simulink model "ddcnco"  (Simulink 6.1)
settings: Solver=FixedStepDiscrete  SolverMode=SingleTasking  StartTime=0.0  StopTime=20544/69.333e6  RelTol=1e-3
values from neighbouring files (symbols this model uses):
  D = [0 : 1/1E3 : 10E-3 ; 0.8.^(0:10)]'    [waveformdemo.m]
libraries: simulink x6, dspsnks4 x1, dspsigops x1, dspindex x1
settings Model: MinMaxOverflowLogging=OverflowOnly  Creator=The MathWorks Inc.  LastModifiedBy=pjp  ExtModeAutoUpdateStatusClock=off  ProdHWDeviceType=ASIC/FPGA
settings DataIOCC: LimitDataPoints=off  SaveOutput=off  SignalLogging=off  SaveTime=off  SignalLoggingName=sigsOut
settings OptimizationCC: InlineParams=on  BufferReusableBoundary=off
settings DebuggingCC: CheckExecutionContextPreStartOutputMsg=on  CheckExecutionContextRuntimeOutputMsg=on  IntegerOverflowMsg=none  ParameterPrecisionLossMsg=none  BusObjectLabelMismatch=off
settings HardwareCC: ProdHWDeviceType=ASIC/FPGA

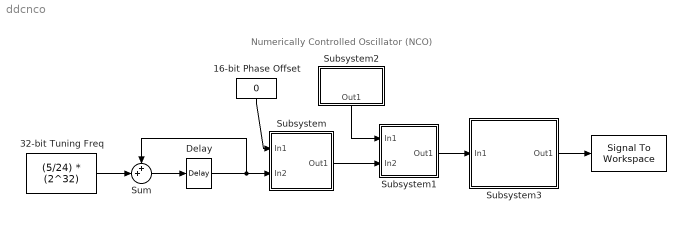
== system ddcnco ==
  note: Numerically Controlled Oscillator (NCO)
  "  " : dspsnks4/Signal To Workspace  VariableName=nco_nodither  FrameMode=Concatenate frames (2-D array)
      settings: AttributesFormatString=\n  Decimation=1  FixptAsFi=off
  16-bit Phase Offset : Constant  Orientation=down  Value=0  OutDataTypeMode=Specify via dialog  OutDataType=ufix(16)  OutScaling=2^-0  SampleTime=1/69.333e6
  32-bit Tuning Freq : Constant  Value=(5/24) * (2^32)  OutDataTypeMode=Specify via dialog  OutDataType=ufix(32)  OutScaling=2^-0  SampleTime=1/69.333e6
  Delay : dspsigops/Delay  dly_unit=Samples  delay=1  ic_detail=off  dif_ic_for_ch=off  dif_ic_for_dly=off  ic=0  reset_popup=None
  Subsystem : Subsystem
      mask Display: disp(['Sum and\nretain\n23 MSBs'])
  Subsystem1 : Subsystem
      mask Display: disp('Sum and\nretain\n18 MSBs')
  Subsystem2 : Subsystem  Orientation=down
      mask Display: disp(['Dither' 10 'Generator'])
  Subsystem3 : Subsystem
      mask Display: disp(['Sine/Cosine\nLookup'])
  Sum : Sum  Inputs=++|  OutDataTypeMode=uint32  RndMeth=Nearest
  wires:
  Delay/1 -> Sum/1, Subsystem/2(In2)
  Sum/1 -> Delay/1
  Subsystem1/1(Out1) -> Subsystem3/1(In1)
  Subsystem3/1(Out1) -> "  "/1
  16-bit Phase Offset/1 -> Subsystem/1(In1)
  Subsystem2/1(Out1) -> Subsystem1/1(In1)
  Subsystem/1(Out1) -> Subsystem1/2(In2)
  32-bit Tuning Freq/1 -> Sum/2

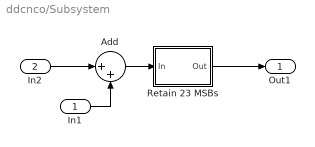
== system ddcnco/Subsystem ==
  In1 : Inport  Port=1  LatchInput=off
  In2 : Inport  Port=2  LatchInput=off
  Add : Sum  Inputs=|++  OutDataTypeMode=Specify via dialog  OutDataType=ufix(32)  OutScaling=2^-0
  Retain 23 MSBs : Subsystem
  Out1 : Outport
  wires:
  Add/1 -> Retain 23 MSBs/1(In)
  Retain 23 MSBs/1(Out) -> Out1/1
  In2/1 -> Add/1
  In1/1 -> Add/2

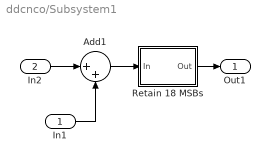
== system ddcnco/Subsystem1 ==
  In1 : Inport  Port=1  LatchInput=off
  In2 : Inport  Port=2  LatchInput=off
  Add1 : Sum  Inputs=|++  OutDataTypeMode=Specify via dialog  OutDataType=ufix(23)  OutScaling=2^-0  InputSameDT=on
  Retain 18 MSBs : Subsystem
  Out1 : Outport
  wires:
  Add1/1 -> Retain 18 MSBs/1(In)
  Retain 18 MSBs/1(Out) -> Out1/1
  In2/1 -> Add1/1
  In1/1 -> Add1/2

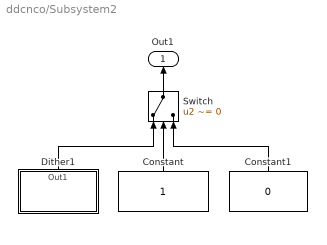
== system ddcnco/Subsystem2 ==
  Constant : Constant  Orientation=up  OutDataTypeMode=boolean
  Constant1 : Constant  Orientation=up  Value=0  OutDataTypeMode=Specify via dialog  OutDataType=ufix(23)
  Dither1 : Subsystem  Orientation=up
      mask Display: disp(['DITHER' 10 'GENERATOR'])
  Switch : Switch  Orientation=up  Criteria=u2 ~= 0  Threshold=0.5  InputSameDT=on
  Out1 : Outport  Orientation=up
  wires:
  Constant/1 -> Switch/2
  Constant1/1 -> Switch/3
  Dither1/1(Out1) -> Switch/1
  Switch/1 -> Out1/1

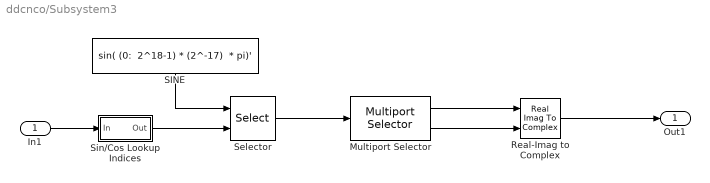
== system ddcnco/Subsystem3 ==
  In1 : Inport  Port=1  LatchInput=off
  Multiport Selector : dspindex/Multiport Selector  rowsOrCols=Rows  idxCellArray={ 1, 2 }  idxErrMode=Clip Index
  Real-Imag to Complex : RealImagToComplex
  SINE : Constant  Orientation=down  Value="sin( (0:  2^18-1) * (2^-17)  * pi)'"  VectorParams1D=off  OutDataTypeMode=Specify via dialog  OutDataType=sfix(20)  OutScaling=2^-18
  Selector : Selector  ElementSrc=External  Elements=[1 3]  InputPortWidth=2^18
  Sin/Cos Lookup Indices : Subsystem
  Out1 : Outport
  wires:
  SINE/1 -> Selector/1
  Sin/Cos Lookup Indices/1(Out) -> Selector/2
  In1/1 -> Sin/Cos Lookup Indices/1(In)
  Selector/1 -> Multiport Selector/1
  Multiport Selector/1 -> Real-Imag to Complex/1
  Multiport Selector/2 -> Real-Imag to Complex/2
  Real-Imag to Complex/1 -> Out1/1

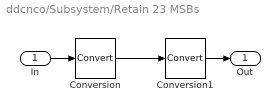
== system ddcnco/Subsystem/Retain 23 MSBs ==
  In : Inport  Port=1  LatchInput=off
  Conversion : DataTypeConversion  OutDataTypeMode=Specify via dialog  OutDataType=ufix(23)  OutScaling=2^9
  Conversion1 : DataTypeConversion  OutDataTypeMode=Specify via dialog  OutDataType=ufix(23)  ConvertRealWorld=Stored Integer (SI)
  Out : Outport
  wires:
  Conversion/1 -> Conversion1/1
  Conversion1/1 -> Out/1
  In/1 -> Conversion/1

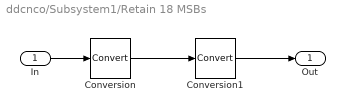
== system ddcnco/Subsystem1/Retain 18 MSBs ==
  In : Inport  Port=1  LatchInput=off
  Conversion : DataTypeConversion  OutDataTypeMode=Specify via dialog  OutDataType=ufix(23)  OutScaling=2^5
  Conversion1 : DataTypeConversion  OutDataTypeMode=Specify via dialog  OutDataType=ufix(18)  ConvertRealWorld=Stored Integer (SI)
  Out : Outport
  wires:
  Conversion/1 -> Conversion1/1
  Conversion1/1 -> Out/1
  In/1 -> Conversion/1

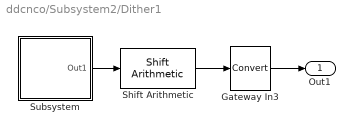
== system ddcnco/Subsystem2/Dither1 ==
  Gateway In3 : DataTypeConversion  OutDataTypeMode=Specify via dialog  OutDataType=ufix(23)
  Shift Arithmetic : simulink/Logic and Bit Operations/Shift Arithmetic  nBitShiftRight=(19-0)  nBinPtShiftRight=0
  Subsystem : Subsystem  mask{nbit=19, ts=1/69.333e6}
      mask prompts: nbit "Shift register size (nbits):"; ts "Sample time:"
      mask Display: disp(['Fixed-point' 10 'Random' 10 'Number' 10 'Generator'])
  Out1 : Outport
  wires:
  Gateway In3/1 -> Out1/1
  Subsystem/1(Out1) -> Shift Arithmetic/1
  Shift Arithmetic/1 -> Gateway In3/1

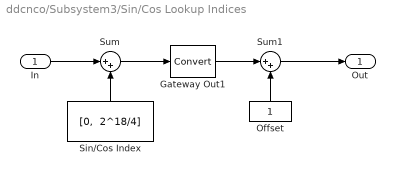
== system ddcnco/Subsystem3/Sin/Cos Lookup Indices ==
  In : Inport  Port=1  LatchInput=off
  Gateway Out1 : DataTypeConversion  OutDataTypeMode=uint32  ConvertRealWorld=Stored Integer (SI)
  Offset : Constant  Orientation=up  OutDataTypeMode=Specify via dialog  OutDataType=uint(32)  OutScaling=2^-0
  Sin/Cos Index : Constant  Orientation=up  Value="[0,  2^18/4]"  OutDataType=sfix(5)  OutScaling=2^-0
  Sum : Sum  Inputs=|++  InputSameDT=on
  Sum1 : Sum  Inputs=|++  InputSameDT=on
  Out : Outport
  wires:
  Sum/1 -> Gateway Out1/1
  In/1 -> Sum/1
  Sin/Cos Index/1 -> Sum/2
  Sum1/1 -> Out/1
  Gateway Out1/1 -> Sum1/1
  Offset/1 -> Sum1/2

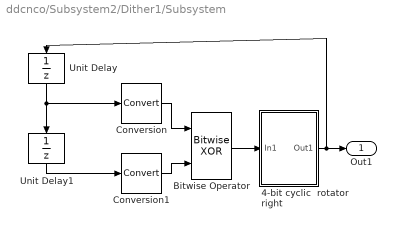
== system ddcnco/Subsystem2/Dither1/Subsystem ==
  4-bit cyclic  rotator right : Subsystem
      mask Display: disp(['Cyclic' 10 'Right' 10 'Rotator' 10 'ROR'])
  Bitwise Operator : simulink/Logic and Bit Operations/Bitwise Operator  logicop=XOR  UseBitMask=off  NumInputPorts=2  BitMask=bin2dec('11011001')  BitMaskRealWorld=Stored Integer
  Conversion : DataTypeConversion  OutDataTypeMode=Specify via dialog  OutDataType=ufix(nbit)
  Conversion1 : DataTypeConversion  OutDataTypeMode=Specify via dialog  OutDataType=ufix(nbit)
  Unit Delay : UnitDelay  Orientation=down  X0=1  SampleTime=ts
  Unit Delay1 : UnitDelay  Orientation=down  X0=2  SampleTime=ts
  Out1 : Outport
  wires:
  Unit Delay1/1 -> Conversion1/1
  Conversion1/1 -> Bitwise Operator/2
  Conversion/1 -> Bitwise Operator/1
  4-bit cyclic  rotator right/1(Out1) -> Unit Delay/1, Out1/1
  Bitwise Operator/1 -> 4-bit cyclic  rotator right/1(In1)
  Unit Delay/1 -> Conversion/1, Unit Delay1/1

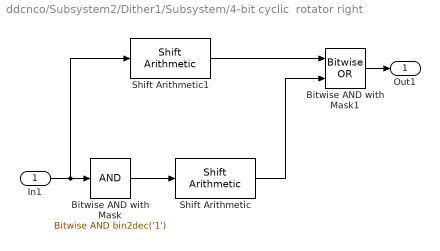
== system ddcnco/Subsystem2/Dither1/Subsystem/4-bit cyclic  rotator right ==
  In1 : Inport  Port=1  LatchInput=off
  Bitwise AND with Mask : simulink/Logic and Bit Operations/Bitwise Operator  logicop=AND  UseBitMask=on  BitMask=bin2dec('1')  BitMaskRealWorld=Stored Integer
  Bitwise AND with Mask1 : simulink/Logic and Bit Operations/Bitwise Operator  logicop=OR  UseBitMask=off  NumInputPorts=2  BitMask=bin2dec('1')  BitMaskRealWorld=Stored Integer
  Shift Arithmetic : simulink/Logic and Bit Operations/Shift Arithmetic  nBitShiftRight=-(nbit-1)  nBinPtShiftRight=0
  Shift Arithmetic1 : simulink/Logic and Bit Operations/Shift Arithmetic  nBitShiftRight=1  nBinPtShiftRight=0
  Out1 : Outport
  wires:
  In1/1 -> Shift Arithmetic1/1, Bitwise AND with Mask/1
  Bitwise AND with Mask/1 -> Shift Arithmetic/1
  Shift Arithmetic/1 -> Bitwise AND with Mask1/2
  Shift Arithmetic1/1 -> Bitwise AND with Mask1/1
  Bitwise AND with Mask1/1 -> Out1/1
